simulink model "mconversion_error"  (Simulink 7.4)
settings: Solver=ode1  StartTime=0.0  StopTime=10.0  FixedStep=0.001  RelTol=1e-3
settings Model: Creator=JUTTAL  LastModifiedBy=mtocci
settings OptimizationCC: InlineParams=on  CVOUCH=off
settings DebuggingCC: StrictBusMsg=ErrorLevel1
settings SFSimCC: SimGenerateEmlReport=off

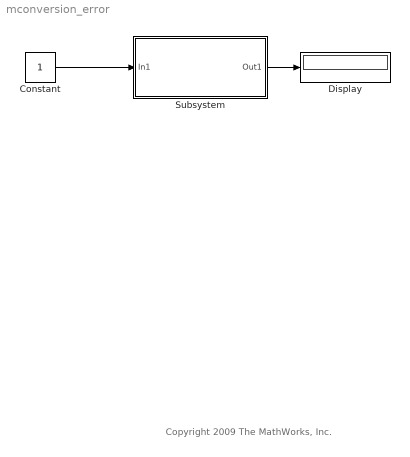
== system mconversion_error ==
  note: Copyright 2009 The MathWorks, Inc.
  Constant : Constant  OutDataType=fixdt(1, 16)  OutScaling=2^0  SampleTime=0.001
  Display : Display
  Subsystem : Subsystem  TreatAsAtomicUnit=on
  wires:
  Constant/1 -> Subsystem/1(In1)
  Subsystem/1(Out1) -> Display/1

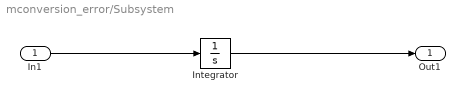
== system mconversion_error/Subsystem ==
  In1 : Inport  PortDimensions=1
  Integrator : Integrator
  Out1 : Outport  PortDimensions=1
  wires:
  Integrator/1 -> Out1/1
  In1/1 -> Integrator/1
